simulink model "GmC2ndCTSDMParam"  (R2022a)
settings: Solver=ode45  StartTime=0.0  StopTime=(N-1)*ts  RelTol=1e-3  EnableMultiTasking=on
model workspace (MATLAB code in the model file):
  | % Load model parameters
  | 
  | Gm2ndCTSDMparameters
undefined symbols (not defined in the file or in its folder): Ain, C1, C2, f11, f12, fin, gm, gm11, gq1, R11, R12, ts, vhigh, vlow
libraries: otaclib x7, quantidlib x1
settings Model: SimulationMode=rapid-accelerator  Creator=Administrador  LastModifiedBy=jrosa
settings SolverCC: ZeroCrossAlgorithm=Non-adaptive  AlgebraicLoopSolver=TrustRegion
settings DataIOCC: LimitDataPoints=on  SaveFormat=Array  SignalLoggingSaveFormat=ModelDataLogs  ReturnWorkspaceOutputs=off
settings OptimizationCC: ExpressionDepthLimit=2147483647  InitFltsAndDblsToZero=on  LifeSpan=inf
settings DebuggingCC: SaveWithParameterizedLinksMsg=none  UnderspecifiedInitializationDetection=Classic  MergeDetectMultiDrivingBlocksExec=none  SignalResolutionControl=TryResolveAllWithWarning  SolverPrmCheckMsg=warning  FcnCallInpInsideContextMsg=warning  UnconnectedInputMsg=warning  UnconnectedOutputMsg=warning  UnconnectedLineMsg=warning  StateNameClashWarn=warning  SFUnexpectedBacktrackingDiag=warning  SFNoUnconditionalDefaultTransitionDiag=warning  SFExecutionAtInitializationDiag=none  SFMachineParentedDataDiag=warning  ArithmeticOperatorsInVariantConditions=warning
settings HardwareCC: ProdBitPerPointer=32  ProdBitPerSizeT=32  ProdBitPerPtrDiffT=32  ProdLargestAtomicFloat=None  ProdIntDivRoundTo=Undefined  ProdEndianess=Unspecified  ProdWordSize=32  ProdHWDeviceType=32-bit Generic
settings ModelReferenceCC: PropagateSignalLabelsOutOfModel=off
settings CodeAppCC: StateflowObjectComments=on
settings GRTTargetCC: TargetFcnLib=ansi_tfl_tmw.mat  TargetLangStandard=C89/C90 (ANSI)  CombineOutputUpdateFcns=off  GRTInterface=on
settings ConfigComp: CovMetricSettings=dw  CovSaveCumulativeToWorkspaceVar=on  CovSaveSingleToWorkspaceVar=on

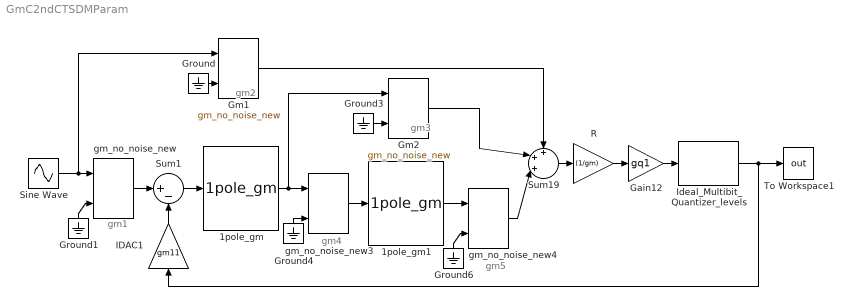
== system GmC2ndCTSDMParam ==
  note: gm2
  note: gm1
  note: gm4
  note: gm3
  note: gm5
  1pole_gm : otaclib/1pole_gm  C=C1  Cp=Cp1  R=R11
  1pole_gm1 : otaclib/1pole_gm  C=C2  Cp=Cp2  R=R12
  Gain12 : Gain  Gain=gq1  SampleTime=0
  Gm1 : otaclib/gm_no_noise_new  GM=gm*fi  IIP3=IIP3_a  MAX_OUT=vos_gm  MAX_IN=vis_gm
  Gm2 : otaclib/gm_no_noise_new  GM=gm*f11  IIP3=IIP3_b  MAX_OUT=vos_gm  MAX_IN=vis_gm
  Ground{,1,3..4,6} (5 alike) : Ground
  IDAC1 : Gain  Gain=gm11  SaturateOnIntegerOverflow=on  SampleTime=0  OutDataTypeStr=Inherit: Same as input  ParamDataTypeStr=Inherit: Same as input
  Ideal_Multibit_Quantizer_levels : quantidlib/Ideal_Multibit_Quantizer_levels  Vhigh=vhigh  Vlow=vlow  n_levels=n_levels  Xfs=(vhigh-vlow)  phi=phi1  ts=ts  qid=q1
      link override Goto: GotoTag=q1
  R : Gain  Gain=(1/gm)  SaturateOnIntegerOverflow=on  SampleTime=0  OutDataTypeStr=Inherit: Same as input  ParamDataTypeStr=Inherit: Same as input
  Sine Wave : Sin  Amplitude=Ain  Frequency=2*pi*fin  SampleTime=0
  Sum1 : Sum  Inputs=|+-  SaturateOnIntegerOverflow=on  SampleTime=0
  Sum19 : Sum  Inputs=+++|  SaturateOnIntegerOverflow=on  SampleTime=0
  To Workspace1 : ToWorkspace  VariableName=out  SampleTime=ts
  gm_no_noise_new : otaclib/gm_no_noise_new  GM=gm11  IIP3=IIP3_in  MAX_OUT=vos_gm  MAX_IN=vis_gm
  gm_no_noise_new3 : otaclib/gm_no_noise_new  GM=gm12  IIP3=IIP3_12  MAX_OUT=vos_gm  MAX_IN=vis_gm
  gm_no_noise_new4 : otaclib/gm_no_noise_new  GM=gm*f12  IIP3=IIP3_c  MAX_OUT=vos_gm  MAX_IN=vis_gm
  wires:
  Ground/1 -> Gm1/2
  gm_no_noise_new/1 -> Sum1/1
  Sum1/1 -> 1pole_gm/1
  1pole_gm/1 -> Gm2/1, gm_no_noise_new3/1
  gm_no_noise_new3/1 -> 1pole_gm1/1
  1pole_gm1/1 -> gm_no_noise_new4/1
  Ground3/1 -> Gm2/2
  Gm2/1 -> Sum19/2
  gm_no_noise_new4/1 -> Sum19/3
  Gm1/1 -> Sum19/1
  Sum19/1 -> R/1
  IDAC1/1 -> Sum1/2
  R/1 -> Gain12/1
  Sine Wave/1 -> gm_no_noise_new/1, Gm1/1
  Ground1/1 -> gm_no_noise_new/2
  Ground4/1 -> gm_no_noise_new3/2
  Ground6/1 -> gm_no_noise_new4/2
  Ideal_Multibit_Quantizer_levels/1 -> IDAC1/1, To Workspace1/1
  Gain12/1 -> Ideal_Multibit_Quantizer_levels/1
